simulink model "filter_test"  (R2016a)
settings: Solver=FixedStepAuto  StartTime=0.0  StopTime=170  FixedStep=0.01  RelTol=1e-3
libraries: dspstat3 x2
settings Model: Creator=Guttorm  LastModifiedBy=Guttorm
settings DataIOCC: LimitDataPoints=on  SaveFormat=Array
settings HardwareCC: ProdBitPerPointer=32  ProdLargestAtomicFloat=None  ProdIntDivRoundTo=Undefined  ProdEndianess=Unspecified  ProdWordSize=32  ProdHWDeviceType=32-bit Generic
settings ModelReferenceCC: PropagateSignalLabelsOutOfModel=off
settings ConfigComp: CovModelRefEnable=Off

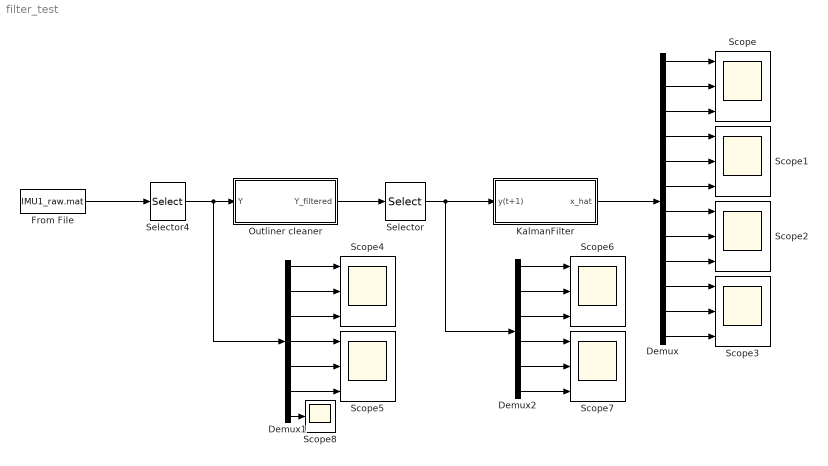
== system filter_test ==
  Demux : Demux  Outputs=12
  Demux1 : Demux  Outputs=7
  Demux2 : Demux  Outputs=6
  From File : FromFile  FileName=IMU1_raw.mat  SampleTime=0.01
  KalmanFilter : Subsystem  mask{Q=10^-6*eye(12), A=[1, 0, 0, 0, 0, 0, 0, 0, 0, 0, 0, 0; 0, 1, 0, 0, 0, 0, 0, 0, 0, 0, 0, 0; 0, 0, 1, 0, 0, 0, 0, 0, 0, 0, 0, 0; 0.01, 0, 0, 1, 0, 0, 0, 0, 0, 0, 0, 0; 0, 0.01, 0, 0, 1, 0, 0, 0, 0, 0, 0, 0; 0, 0, 0.01, 0, 0, 1, 0, 0, 0, 0, 0, 0; 0, 0, 0, 0, 0, 0, 1, 0, 0, 0, 0, 0; 0, 0, 0, 0, 0, 0, 0, 1, 0, 0, 0, 0; 0, 0, 0, 0, 0, 0, 0, 0, 1, 0, 0, 0; 0, 0, 0, 0, 0, 0, 0.01, 0, 0, 1, 0, 0; 0, 0, 0, 0, 0, 0, 0, 0.01, 0, 0, 1, 0; 0, 0, 0, 0, 0, 0, 0, 0, 0.01, 0, 0, 1], H=[1, 0, 0, 0, 0, 0, 0, 0, 0, 0, 0, 0; 0, 1, 0, 0, 0, 0, 0, 0, 0, 0, 0, 0; 0, 0, 1, 0, 0, 0, 0, 0, 0, 0, 0, 0; 0, 0, 0, 0, 0, 0, 1, 0, 0, 0, 0, 0; 0, 0, 0, 0, 0, 0, 0, 1, 0, 0, 0, 0; 0, 0, 0, 0, 0, 0, 0, 0, 1, 0, 0, 0], R=diag([0.1102, 0.1058, 0.1206, 4.9686, 4.2253, 4.1697])}
  Outliner cleaner : Subsystem
  Scope{,1..7} (8 alike) : Scope  NumInputPorts=3
  Scope8 : Scope
  Selector : Selector  InputPortWidth=7  IndexOptions=Index vector (dialog)  Indices=[1:6]  OutputSizes=1
  Selector4 : Selector  InputPortWidth=7  IndexOptions=Index vector (dialog)  Indices=[1:7]  OutputSizes=1
  wires:
  Outliner cleaner/1(Y_filtered) -> Selector/1
  KalmanFilter/1(x_hat) -> Demux/1
  From File/1 -> Selector4/1
  Demux/1 -> Scope/1
  Demux/2 -> Scope/2
  Demux/3 -> Scope/3
  Demux/5 -> Scope1/2
  Demux/6 -> Scope1/3
  Demux/4 -> Scope1/1
  Demux/8 -> Scope2/2
  Demux/9 -> Scope2/3
  Demux/7 -> Scope2/1
  Demux/12 -> Scope3/3
  Demux/11 -> Scope3/2
  Demux/10 -> Scope3/1
  Selector4/1 -> Demux1/1, Outliner cleaner/1(Y)
  Demux1/1 -> Scope4/1
  Demux1/2 -> Scope4/2
  Demux1/3 -> Scope4/3
  Demux1/5 -> Scope5/2
  Demux1/6 -> Scope5/3
  Demux1/4 -> Scope5/1
  Demux1/7 -> Scope8/1
  Selector/1 -> Demux2/1, KalmanFilter/1(y(t+1))
  Demux2/1 -> Scope6/1
  Demux2/2 -> Scope6/2
  Demux2/3 -> Scope6/3
  Demux2/5 -> Scope7/2
  Demux2/6 -> Scope7/3
  Demux2/4 -> Scope7/1

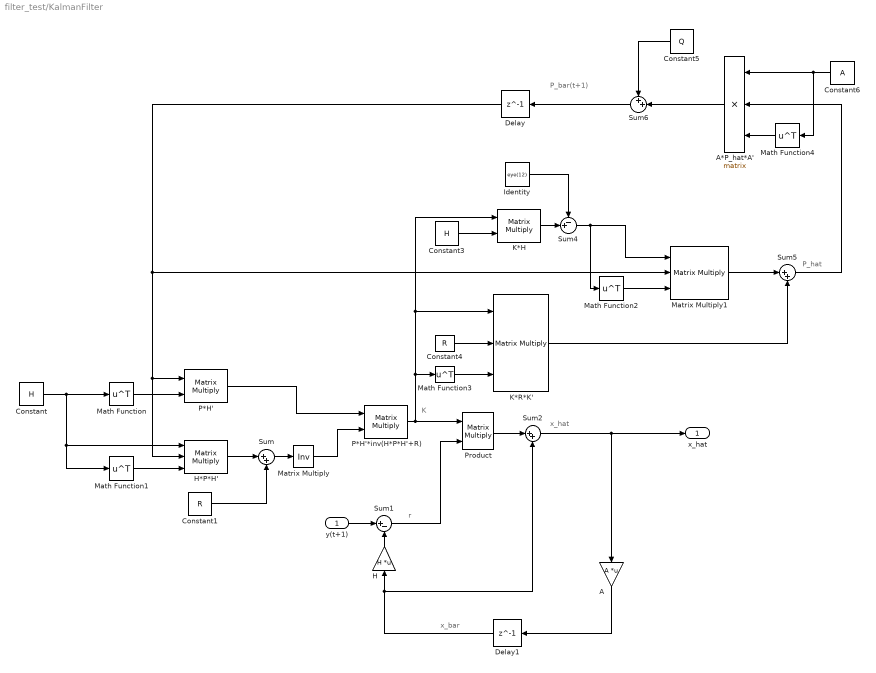
== system filter_test/KalmanFilter ==
  note: P_bar(t+1)
  note: P_hat
  note: x_hat
  note: x_bar
  note: r
  note: K
  y(t+1) : Inport
  A : Gain  Gain=A  Multiplication=Matrix(K*u)
  A*P_hat*A' : Product  Inputs=3  Multiplication=Matrix(*)
  Constant : Constant  Value=H
  Constant1 : Constant  Value=R
  Constant3 : Constant  Value=H
  Constant4 : Constant  Value=R
  Constant5 : Constant  Value=Q
  Constant6 : Constant  Value=A
  Delay : Delay  DelayLength=1  InitialCondition=eye(12)
  Delay1 : Delay  DelayLength=1  InitialCondition=[0 0 0 0 0 0 0 0 0 0 0 0]
  H : Gain  Gain=H  Multiplication=Matrix(K*u)
  H*P*H' : Product  Inputs=3  Multiplication=Matrix(*)
  Identity : Constant  Value=eye(12)
  K*H : Product  Multiplication=Matrix(*)
  K*R*K' : Product  Inputs=3  Multiplication=Matrix(*)
  Math Function{,1..4} (5 alike) : Math  Operator=transpose  SaturateOnIntegerOverflow=on
  Matrix Multiply : Product  Inputs=/  Multiplication=Matrix(*)
  Matrix Multiply1 : Product  Inputs=3  Multiplication=Matrix(*)
  P*H' : Product  Multiplication=Matrix(*)
  P*H'*inv(H*P*H'+R) : Product  Multiplication=Matrix(*)
  Product : Product  Multiplication=Matrix(*)
  Sum : Sum  Inputs=|++
  Sum1 : Sum  Inputs=|+-
  Sum2 : Sum  Inputs=|++
  Sum4 : Sum  Inputs=-+|
  Sum5 : Sum  Inputs=|++
  Sum6 : Sum  Inputs=++|
  x_hat : Outport
  wires:
  Constant/1 -> Math Function1/1, H*P*H'/1, Math Function/1
  Math Function/1 -> P*H'/2
  Math Function1/1 -> H*P*H'/3
  H*P*H'/1 -> Sum/1
  Constant1/1 -> Sum/2
  Sum/1 -> Matrix Multiply/1
  Matrix Multiply/1 -> P*H'*inv(H*P*H'+R)/2
  P*H'/1 -> P*H'*inv(H*P*H'+R)/1
  y(t+1)/1 -> Sum1/1
  H/1 -> Sum1/2
  Delay1/1 -> Sum2/2, H/1
  Sum1/1 -> Product/2
  P*H'*inv(H*P*H'+R)/1 -> K*H/1, K*R*K'/1, Math Function3/1, Product/1
  Product/1 -> Sum2/1
  Sum2/1 -> A/1, x_hat/1
  A/1 -> Delay1/1
  Identity/1 -> Sum4/1
  K*H/1 -> Sum4/2
  Constant3/1 -> K*H/2
  Sum4/1 -> Math Function2/1, Matrix Multiply1/1
  Math Function2/1 -> Matrix Multiply1/3
  Constant4/1 -> K*R*K'/2
  Math Function3/1 -> K*R*K'/3
  K*R*K'/1 -> Sum5/2
  Matrix Multiply1/1 -> Sum5/1
  Sum5/1 -> A*P_hat*A'/2
  Sum6/1 -> Delay/1
  Constant5/1 -> Sum6/1
  A*P_hat*A'/1 -> Sum6/2
  Constant6/1 -> Math Function4/1, A*P_hat*A'/1
  Math Function4/1 -> A*P_hat*A'/3
  Delay/1 -> H*P*H'/2, P*H'/1, Matrix Multiply1/2

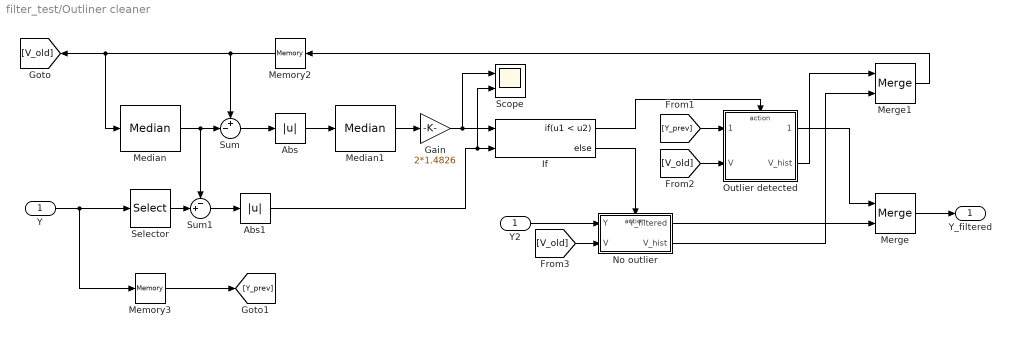
== system filter_test/Outliner cleaner ==
  Y : Inport
  Abs : Abs
  Abs1 : Abs
  Gain : Gain  Gain=2*1.4826
  If : If  NumInputs=2  IfExpression=u1 < u2
  Median : dspstat3/Median  sortAlg=Quick sort  directionMode=Entire input  dimension=1  outputDataTypeStr=Inherit: Same as accumulator  outputLastDataTypeStr=Inherit: Same as accumulator  outputMin=[]  outputMax=[]  accumDataTypeStr=Inherit: Same as product output  accumLastDataTypeStr=Inherit: Same as product output  roundingMode=Floor  overflowMode=off
      settings: allowOverrides=off
  Median1 : dspstat3/Median  sortAlg=Quick sort  directionMode=Entire input  dimension=1  outputDataTypeStr=Inherit: Same as accumulator  outputLastDataTypeStr=Inherit: Same as accumulator  outputMin=[]  outputMax=[]  accumDataTypeStr=Inherit: Same as product output  accumLastDataTypeStr=Inherit: Same as product output  roundingMode=Floor  overflowMode=off
      settings: allowOverrides=off
  Memory2 : Memory  X0=[4.968, 4.965, 4.97, 4.975, 4.96]
  Memory3 : Memory  X0=[0, 0, 0, 0, 0, 0, 0]
  Merge : Merge
  Merge1 : Merge
  No outlier : Subsystem  TreatAsAtomicUnit=on
  Outlier detected : Subsystem  TreatAsAtomicUnit=on
  Scope : Scope  NumInputPorts=2
  Selector : Selector  InputPortWidth=7  IndexOptions=Index vector (dialog)  Indices=[7]  OutputSizes=1
  Sum : Sum  Inputs=+-|
  Sum1 : Sum  Inputs=-+|
  Y2 : InportShadow
  Y_filtered : Outport
  wires:
  Memory2/1 -> Sum/1, [V_old], Median/1
  Median/1 -> Sum1/1, Sum/2
  Sum/1 -> Abs/1
  Abs/1 -> Median1/1
  Y/1 -> Memory3/1, Selector/1
  Selector/1 -> Sum1/2
  Sum1/1 -> Abs1/1
  Abs1/1 -> Scope/2, If/2
  Gain/1 -> Scope/1, If/1
  [Y_prev] -> Outlier detected/1(Y_previous)
  Outlier detected/1(Y_filtered) -> Merge/1
  If/1 -> Outlier detected/Action
  If/2 -> No outlier/Action
  Y2/1 -> No outlier/1(Y)
  Merge1/1 -> Memory2/1
  No outlier/1(Y_filtered) -> Merge/2
  Median1/1 -> Gain/1
  Memory3/1 -> [Y_prev]
  Merge/1 -> Y_filtered/1
  [V_old] -> Outlier detected/2(V)
  Outlier detected/2(V_hist) -> Merge1/1
  [V_old] -> No outlier/2(V)
  No outlier/2(V_hist) -> Merge1/2

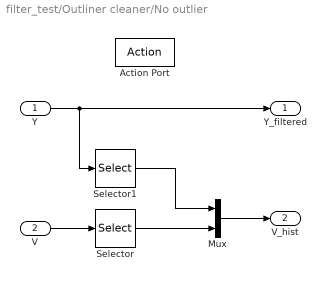
== system filter_test/Outliner cleaner/No outlier ==
  Y : Inport
  V : Inport  Port=2
  Action Port : ActionPort  ActionType=else
  Mux : Mux  Inputs=2
  Selector : Selector  InputPortWidth=5  IndexOptions=Index vector (dialog)  Indices=[2:5]  OutputSizes=1
  Selector1 : Selector  InputPortWidth=7  IndexOptions=Index vector (dialog)  Indices=[7]  OutputSizes=1
  Y_filtered : Outport
  V_hist : Outport  Port=2
  wires:
  Y/1 -> Selector1/1, Y_filtered/1
  V/1 -> Selector/1
  Selector/1 -> Mux/2
  Selector1/1 -> Mux/1
  Mux/1 -> V_hist/1

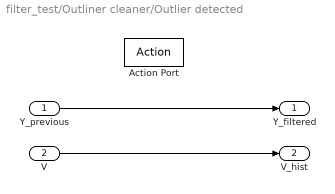
== system filter_test/Outliner cleaner/Outlier detected ==
  Y_previous : Inport
  V : Inport  Port=2
  Action Port : ActionPort  ActionType=then
  Y_filtered : Outport
  V_hist : Outport  Port=2
  wires:
  Y_previous/1 -> Y_filtered/1
  V/1 -> V_hist/1
